simulink model "A1"  (R2023b)
settings: Solver=FixedStepAuto  StartTime=0.0  StopTime=10  FixedStep=1e-3  RelTol=1e-3  EnableMultiTasking=on
undefined symbols (not defined in the file or in its folder): D0, D1, D10, D11, D12, D13, D2, D3, D4, D5, D6, D7, D8, D9, PTA0, PTA1, PTA2, PTB23, PTB9, PTC16, PTC17, PTC2, PTC3, PTC4, PTD0, PTD1, PTD2, PTD3
libraries: frdmk64flib x15
settings Model: PacingRate=0.250000  ExtModeTrigDuration=5  Creator=mathewgaluszka  LastModifiedBy=himan
settings OptimizationCC: EnhancedBackFolding=on  PassReuseOutputArgsAs=Individual arguments  ZeroExternalMemoryAtStartup=off  ZeroInternalMemoryAtStartup=off  MaxStackSize=64  OptimizeBlockOrder=speed  DifferentSizesBufferReuse=on  OptimizationCustomize=off  EfficientTunableParamExpr=on
settings DebuggingCC: ParameterTunabilityLossMsg=error
settings HardwareCC: ProdBitPerPointer=32  ProdBitPerSizeT=32  ProdBitPerPtrDiffT=32  ProdLargestAtomicInteger=Long  ProdLargestAtomicFloat=Double  ProdWordSize=32  ProdHWDeviceType=ARM Compatible->ARM Cortex
settings SFSimCC: MATLABDynamicMemAlloc=off
settings RTWCC: Description=Embedded Coder  SystemTargetFile=ert.tlc  HardwareBoard=NXP FRDM-K64F  TLCOptions="-aInlineSetEventsForThisBaseRateFcn=TLC_FALSE -aSuppressMultiTaskScheduler=TLC_FALSE  -aRateBasedStepFcn=0"  TemplateMakefile=ert_default_tmf  Toolchain=GNU Tools for ARM Embedded Processors
settings CodeAppCC: ForceParamTrailComments=on  IgnoreCustomStorageClasses=off  OperatorAnnotations=on  SimulinkDataObjDesc=on  SFDataObjDesc=on  InsertBlockDesc=on
settings ERTTargetCC: SupportContinuousTime=on  ExtModeTransport=4  ExtModeMexFile=sendToCommService

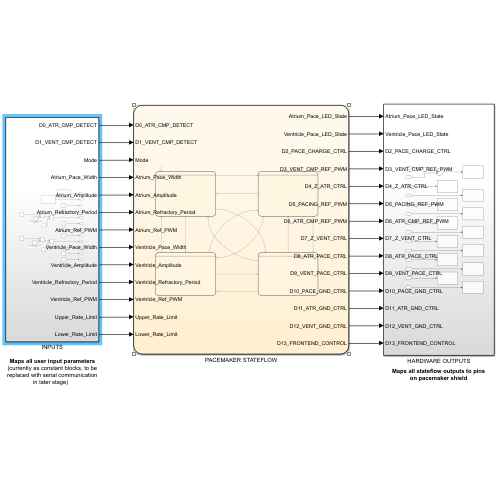
[thumbnail: Simulink's stored preview of the top-level diagram]
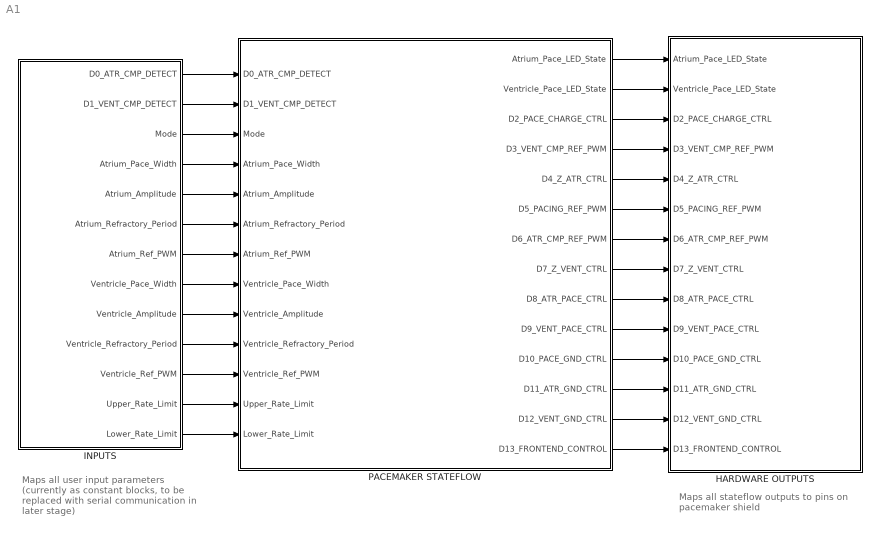
== system A1 ==
  note: Maps all user input parameters (currently as constant blocks, to be replaced with serial communication in later stage)
  note: Maps all stateflow outputs to pins on pacemaker shield
  HARDWARE OUTPUTS : Subsystem
  INPUTS : Subsystem
  PACEMAKER STATEFLOW : Stateflow chart  TreatAsAtomicUnit=on
  wires:
  PACEMAKER STATEFLOW/1(Atrium_Pace_LED_State) -> HARDWARE OUTPUTS/1(Atrium_Pace_LED_State)
  PACEMAKER STATEFLOW/2(Ventricle_Pace_LED_State) -> HARDWARE OUTPUTS/2(Ventricle_Pace_LED_State)
  PACEMAKER STATEFLOW/3(D2_PACE_CHARGE_CTRL) -> HARDWARE OUTPUTS/3(D2_PACE_CHARGE_CTRL)
  PACEMAKER STATEFLOW/4(D3_VENT_CMP_REF_PWM) -> HARDWARE OUTPUTS/4(D3_VENT_CMP_REF_PWM)
  PACEMAKER STATEFLOW/5(D4_Z_ATR_CTRL) -> HARDWARE OUTPUTS/5(D4_Z_ATR_CTRL)
  PACEMAKER STATEFLOW/6(D5_PACING_REF_PWM) -> HARDWARE OUTPUTS/6(D5_PACING_REF_PWM)
  PACEMAKER STATEFLOW/7(D6_ATR_CMP_REF_PWM) -> HARDWARE OUTPUTS/7(D6_ATR_CMP_REF_PWM)
  PACEMAKER STATEFLOW/8(D7_Z_VENT_CTRL) -> HARDWARE OUTPUTS/8(D7_Z_VENT_CTRL)
  PACEMAKER STATEFLOW/9(D8_ATR_PACE_CTRL) -> HARDWARE OUTPUTS/9(D8_ATR_PACE_CTRL)
  PACEMAKER STATEFLOW/10(D9_VENT_PACE_CTRL) -> HARDWARE OUTPUTS/10(D9_VENT_PACE_CTRL)
  PACEMAKER STATEFLOW/11(D10_PACE_GND_CTRL) -> HARDWARE OUTPUTS/11(D10_PACE_GND_CTRL)
  PACEMAKER STATEFLOW/12(D11_ATR_GND_CTRL) -> HARDWARE OUTPUTS/12(D11_ATR_GND_CTRL)
  PACEMAKER STATEFLOW/13(D12_VENT_GND_CTRL) -> HARDWARE OUTPUTS/13(D12_VENT_GND_CTRL)
  PACEMAKER STATEFLOW/14(D13_FRONTEND_CONTROL) -> HARDWARE OUTPUTS/14(D13_FRONTEND_CONTROL)
  INPUTS/1(D0_ATR_CMP_DETECT) -> PACEMAKER STATEFLOW/1(D0_ATR_CMP_DETECT)
  INPUTS/2(D1_VENT_CMP_DETECT) -> PACEMAKER STATEFLOW/2(D1_VENT_CMP_DETECT)
  INPUTS/3(Mode) -> PACEMAKER STATEFLOW/3(Mode)
  INPUTS/4(Atrium_Pace_Width) -> PACEMAKER STATEFLOW/4(Atrium_Pace_Width)
  INPUTS/5(Atrium_Amplitude) -> PACEMAKER STATEFLOW/5(Atrium_Amplitude)
  INPUTS/6(Atrium_Refractory_Period) -> PACEMAKER STATEFLOW/6(Atrium_Refractory_Period)
  INPUTS/7(Atrium_Ref_PWM) -> PACEMAKER STATEFLOW/7(Atrium_Ref_PWM)
  INPUTS/8(Ventricle_Pace_Width) -> PACEMAKER STATEFLOW/8(Ventricle_Pace_Width)
  INPUTS/9(Ventricle_Amplitude) -> PACEMAKER STATEFLOW/9(Ventricle_Amplitude)
  INPUTS/10(Ventricle_Refractory_Period) -> PACEMAKER STATEFLOW/10(Ventricle_Refractory_Period)
  INPUTS/11(Ventricle_Ref_PWM) -> PACEMAKER STATEFLOW/11(Ventricle_Ref_PWM)
  INPUTS/12(Upper_Rate_Limit) -> PACEMAKER STATEFLOW/12(Upper_Rate_Limit)
  INPUTS/13(Lower_Rate_Limit) -> PACEMAKER STATEFLOW/13(Lower_Rate_Limit)

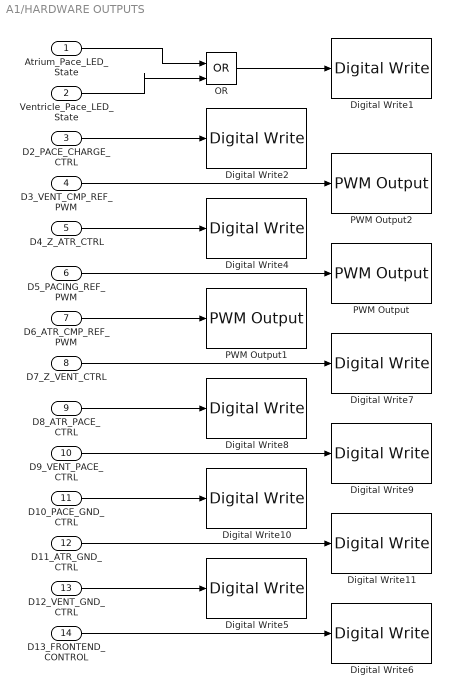
== system A1/HARDWARE OUTPUTS ==
  Atrium_Pace_LED_State : Inport
  Ventricle_Pace_LED_State : Inport  Port=2
  D2_PACE_CHARGE_CTRL : Inport  Port=3
  D3_VENT_CMP_REF_PWM : Inport  Port=4
  D4_Z_ATR_CTRL : Inport  Port=5
  D5_PACING_REF_PWM : Inport  Port=6
  D6_ATR_CMP_REF_PWM : Inport  Port=7
  D7_Z_VENT_CTRL : Inport  Port=8
  D8_ATR_PACE_CTRL : Inport  Port=9
  D9_VENT_PACE_CTRL : Inport  Port=10
  D10_PACE_GND_CTRL : Inport  Port=11
  D11_ATR_GND_CTRL : Inport  Port=12
  D12_VENT_GND_CTRL : Inport  Port=13
  D13_FRONTEND_CONTROL : Inport  Port=14
  Digital Write1 : frdmk64flib/Digital Write  Whichpin=RED_LED
  Digital Write10 : frdmk64flib/Digital Write  Whichpin=PTD0 (D10)
  Digital Write11 : frdmk64flib/Digital Write  Whichpin=PTD2 (D11)
  Digital Write2 : frdmk64flib/Digital Write  Whichpin=PTB9 (D2)
  Digital Write4 : frdmk64flib/Digital Write  Whichpin=PTB23 (D4)
  Digital Write5 : frdmk64flib/Digital Write  Whichpin=PTD3 (D12)
  Digital Write6 : frdmk64flib/Digital Write  Whichpin=PTD1 (D13)
  Digital Write7 : frdmk64flib/Digital Write  Whichpin=PTC3 (D7)
  Digital Write8 : frdmk64flib/Digital Write  Whichpin=PTA0 (D8)
  Digital Write9 : frdmk64flib/Digital Write  Whichpin=PTC4 (D9)
  OR : Logic  Operator=OR  IconShape=distinctive  AllPortsSameDT=off  OutDataTypeStr=boolean
  PWM Output : frdmk64flib/PWM Output  Whichpin=PTA2 (D5)  InitialFrequency=2000  InitialDutyCycle=0
  PWM Output1 : frdmk64flib/PWM Output  Whichpin=PTC2 (D6)  InitialFrequency=2000  InitialDutyCycle=0
  PWM Output2 : frdmk64flib/PWM Output  Whichpin=PTA1 (D3)  InitialFrequency=2000  InitialDutyCycle=0
  wires:
  D2_PACE_CHARGE_CTRL/1 -> Digital Write2/1
  D3_VENT_CMP_REF_PWM/1 -> PWM Output2/1
  D4_Z_ATR_CTRL/1 -> Digital Write4/1
  D5_PACING_REF_PWM/1 -> PWM Output/1
  D6_ATR_CMP_REF_PWM/1 -> PWM Output1/1
  D7_Z_VENT_CTRL/1 -> Digital Write7/1
  D8_ATR_PACE_CTRL/1 -> Digital Write8/1
  D9_VENT_PACE_CTRL/1 -> Digital Write9/1
  D10_PACE_GND_CTRL/1 -> Digital Write10/1
  D11_ATR_GND_CTRL/1 -> Digital Write11/1
  D12_VENT_GND_CTRL/1 -> Digital Write5/1
  D13_FRONTEND_CONTROL/1 -> Digital Write6/1
  Atrium_Pace_LED_State/1 -> OR/1
  Ventricle_Pace_LED_State/1 -> OR/2
  OR/1 -> Digital Write1/1

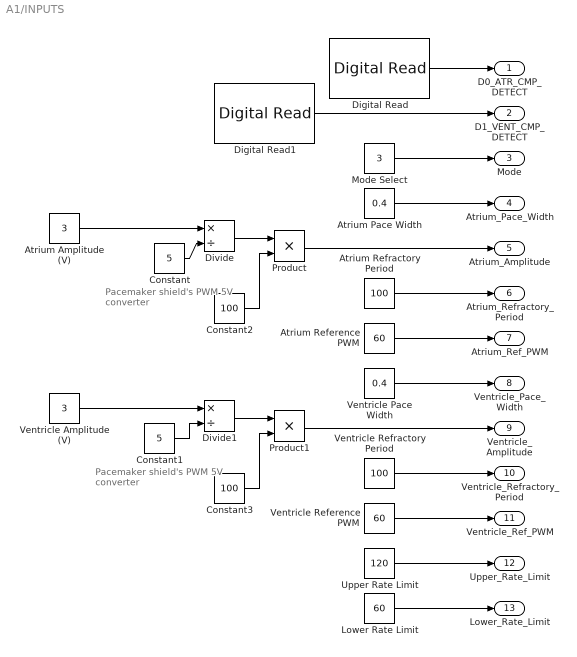
== system A1/INPUTS ==
  note: Pacemaker shield's PWM 5V converter
  note: Pacemaker shield's PWM 5V converter
  Atrium Amplitude (V) : Constant  Value=3
  Atrium Pace Width : Constant  Value=0.4
  Atrium Reference PWM : Constant  Value=60
  Atrium Refractory Period : Constant  Value=100
  Constant : Constant  Value=5
  Constant1 : Constant  Value=5
  Constant2 : Constant  Value=100
  Constant3 : Constant  Value=100
  Digital Read : frdmk64flib/Digital Read  Whichpin=PTC16 (D0)  SampleTime=-1
  Digital Read1 : frdmk64flib/Digital Read  Whichpin=PTC17 (D1)  SampleTime=-1
  Divide : Product  Inputs=*/
  Divide1 : Product  Inputs=*/
  Lower Rate Limit : Constant  Value=60
  Mode Select : Constant  Value=3
  Product : Product
  Product1 : Product
  Upper Rate Limit : Constant  Value=120
  Ventricle Amplitude (V) : Constant  Value=3
  Ventricle Pace Width : Constant  Value=0.4
  Ventricle Reference PWM : Constant  Value=60
  Ventricle Refractory Period : Constant  Value=100
  D0_ATR_CMP_DETECT : Outport
  D1_VENT_CMP_DETECT : Outport  Port=2
  Mode : Outport  Port=3
  Atrium_Pace_Width : Outport  Port=4
  Atrium_Amplitude : Outport  Port=5
  Atrium_Refractory_Period : Outport  Port=6
  Atrium_Ref_PWM : Outport  Port=7
  Ventricle_Pace_Width : Outport  Port=8
  Ventricle_Amplitude : Outport  Port=9
  Ventricle_Refractory_Period : Outport  Port=10
  Ventricle_Ref_PWM : Outport  Port=11
  Upper_Rate_Limit : Outport  Port=12
  Lower_Rate_Limit : Outport  Port=13
  wires:
  Digital Read/1 -> D0_ATR_CMP_DETECT/1
  Digital Read1/1 -> D1_VENT_CMP_DETECT/1
  Mode Select/1 -> Mode/1
  Atrium Pace Width/1 -> Atrium_Pace_Width/1
  Atrium Refractory Period/1 -> Atrium_Refractory_Period/1
  Atrium Reference PWM/1 -> Atrium_Ref_PWM/1
  Ventricle Pace Width/1 -> Ventricle_Pace_Width/1
  Ventricle Refractory Period/1 -> Ventricle_Refractory_Period/1
  Ventricle Reference PWM/1 -> Ventricle_Ref_PWM/1
  Upper Rate Limit/1 -> Upper_Rate_Limit/1
  Lower Rate Limit/1 -> Lower_Rate_Limit/1
  Atrium Amplitude (V)/1 -> Divide/1
  Constant/1 -> Divide/2
  Ventricle Amplitude (V)/1 -> Divide1/1
  Constant1/1 -> Divide1/2
  Divide/1 -> Product/1
  Product/1 -> Atrium_Amplitude/1
  Constant2/1 -> Product/2
  Divide1/1 -> Product1/1
  Product1/1 -> Ventricle_Amplitude/1
  Constant3/1 -> Product1/2

== stateflow chart A1/PACEMAKER STATEFLOW ==
  state AOO
    state Pace
      entry:
      D5_PACING_REF_PWM = 0
      D2_PACE_CHARGE_CTRL=0;
      D10_PACE_GND_CTRL=1;
      D8_ATR_PACE_CTRL=1;
      D11_ATR_GND_CTRL=0;
      D4_Z_ATR_CTRL=0;
      D7_Z_VENT_CTRL=0;
      D12_VENT_GND_CTRL=0;
      D9_VENT_PACE_CTRL=0;
      Atrium_Pace_LED_State=1;
    state Refractory
      entry:
      D10_PACE_GND_CTRL=1;
      D9_VENT_PACE_CTRL=0;
      D4_Z_ATR_CTRL=0;
      D7_Z_VENT_CTRL=0;
      D8_ATR_PACE_CTRL=0;
      D11_ATR_GND_CTRL=1;
      D12_VENT_GND_CTRL=0;
      D2_PACE_CHARGE_CTRL=1;
      D5_PACING_REF_PWM = Atrium_Amplitude
      Atrium_Pace_LED_State=0;
      Standby_Period=(1/(Lower_Rate_Limit))*60000
    (default) -> AOO.Refractory
    AOO.Pace -> AOO.Refractory : [after(Atrium_Pace_Width,msec)]
    AOO.Refractory -> AOO.Pace : [after(Standby_Period,msec)]
  state AAI
    state Refractory
      entry:
      D5_PACING_REF_PWM = Atrium_Amplitude
      D10_PACE_GND_CTRL=1;
      D9_VENT_PACE_CTRL=0;
      D4_Z_ATR_CTRL=0;
      D7_Z_VENT_CTRL=0;
      D8_ATR_PACE_CTRL=0;
      D11_ATR_GND_CTRL=1;
      D12_VENT_GND_CTRL=0;
      D2_PACE_CHARGE_CTRL=1;
      D6_ATR_CMP_REF_PWM = Atrium_Ref_PWM;
      Atrium_Pace_LED_State=0;
      Standby_Period=(1/(Lower_Rate_Limit))*60000-Atrium_Refractory_Period
    state Pace
      entry:
      D5_PACING_REF_PWM = 0
      D2_PACE_CHARGE_CTRL=0;
      D10_PACE_GND_CTRL=1;
      D8_ATR_PACE_CTRL=1;
      D11_ATR_GND_CTRL=0;
      D4_Z_ATR_CTRL=0;
      D7_Z_VENT_CTRL=0;
      D12_VENT_GND_CTRL=0;
      D9_VENT_PACE_CTRL=0;
      Atrium_Pace_LED_State=1;
    (default) -> AAI.Refractory
    AAI.Pace -> (junction 213) : [after(Atrium_Pace_Width,msec)]
    (junction 213) -> AAI.Refractory
    AAI.Refractory -> (junction 213) [order 1] : [D0_ATR_CMP_DETECT == 1]
    (junction 200) -> AAI.Pace [order 2] : after(Standby_Period,msec)
    AAI.Refractory -> (junction 200) [order 2] : [after(Atrium_Refractory_Period,msec) && D0_ATR_CMP_DETECT == 0 ]
    (junction 200) -> AAI.Refractory [order 1] : [D0_ATR_CMP_DETECT == 1]
  state VOO
    state Pace
      entry:
      D5_PACING_REF_PWM = 0
      D2_PACE_CHARGE_CTRL=0;
      D10_PACE_GND_CTRL=1;
      D8_ATR_PACE_CTRL=0;
      D11_ATR_GND_CTRL=0;
      D4_Z_ATR_CTRL=0;
      D7_Z_VENT_CTRL=0;
      D12_VENT_GND_CTRL=0;
      D9_VENT_PACE_CTRL=1;
      Ventricle_Pace_LED_State=1;
    state Refractory
      entry:
      D10_PACE_GND_CTRL=1;
      D9_VENT_PACE_CTRL=0;
      D4_Z_ATR_CTRL=0;
      D7_Z_VENT_CTRL=0;
      D8_ATR_PACE_CTRL=0;
      D11_ATR_GND_CTRL=0;
      D12_VENT_GND_CTRL=1;
      D2_PACE_CHARGE_CTRL=1;
      D5_PACING_REF_PWM = Ventricle_Amplitude
      Ventricle_Pace_LED_State=0;
      Standby_Period=(1/(Lower_Rate_Limit))*60000
    (default) -> VOO.Refractory
    VOO.Pace -> VOO.Refractory : [after(Ventricle_Pace_Width,msec)]
    VOO.Refractory -> VOO.Pace : [after(Standby_Period,msec)]
  state VVI
    state Pace
      entry:
      D5_PACING_REF_PWM = 0
      D2_PACE_CHARGE_CTRL=0;
      D10_PACE_GND_CTRL=1;
      D8_ATR_PACE_CTRL=0;
      D11_ATR_GND_CTRL=0;
      D4_Z_ATR_CTRL=0;
      D7_Z_VENT_CTRL=0;
      D12_VENT_GND_CTRL=0;
      D9_VENT_PACE_CTRL=1;
    state Refractory
      entry:
      D5_PACING_REF_PWM = Ventricle_Amplitude
      D10_PACE_GND_CTRL=1;
      D9_VENT_PACE_CTRL=0;
      D4_Z_ATR_CTRL=0;
      D7_Z_VENT_CTRL=0;
      D8_ATR_PACE_CTRL=0;
      D11_ATR_GND_CTRL=0;
      D12_VENT_GND_CTRL=1;
      D2_PACE_CHARGE_CTRL=1;
      D3_VENT_CMP_REF_PWM = Ventricle_Ref_PWM;
      Ventricle_Pace_LED_State=0;
      Standby_Period=(1/(Lower_Rate_Limit))*60000-Ventricle_Refractory_Period
    (junction 218) -> VVI.Refractory
    VVI.Pace -> (junction 218) : [after(Ventricle_Pace_Width,msec)]
    VVI.Refractory -> (junction 218) [order 1] : [D1_VENT_CMP_DETECT == 1]
    (default) -> VVI.Refractory
    VVI.Refractory -> (junction 219) [order 2] : [after(Ventricle_Refractory_Period,msec) && D1_VENT_CMP_DETECT == 0 ]
    (junction 219) -> VVI.Pace [order 2] : after(Standby_Period,msec)
    (junction 219) -> VVI.Refractory [order 1] : [D1_VENT_CMP_DETECT == 1]
  (default) -> AOO
  AOO -> AAI [order 1] : [Mode==2]
  AAI -> AOO [order 2] : [Mode==0]
  AOO -> VVI [order 3] : [Mode==3]
  VOO -> AAI [order 3] : [Mode==2]
  VOO -> AOO [order 1] : [Mode==0]
  AOO -> VOO [order 2] : [Mode==1]
  VVI -> AOO [order 3] : [Mode==0]
  AAI -> VOO [order 3] : [Mode==1]
  VVI -> AAI [order 2] : [Mode==2]
  AAI -> VVI [order 1] : [Mode==3]
  VOO -> VVI [order 2] : [Mode==3]
  VVI -> VOO [order 1] : [Mode==1]
  data: D0_ATR_CMP_DETECT input; D1_VENT_CMP_DETECT input; Mode input; Atrium_Pace_Width input; Atrium_Amplitude input; Atrium_Refractory_Period input; Atrium_Ref_PWM input; Ventricle_Pace_Width input; Ventricle_Amplitude input; Ventricle_Refractory_Period input; Ventricle_Ref_PWM input; Atrium_Pace_LED_State output; Ventricle_Pace_LED_State output; D2_PACE_CHARGE_CTRL output; D3_VENT_CMP_REF_PWM output; D4_Z_ATR_CTRL output; D5_PACING_REF_PWM output; D6_ATR_CMP_REF_PWM output; D7_Z_VENT_CTRL output; D8_ATR_PACE_CTRL output; D9_VENT_PACE_CTRL output; D10_PACE_GND_CTRL output; D11_ATR_GND_CTRL output; D12_VENT_GND_CTRL output; Upper_Rate_Limit input; Lower_Rate_Limit input; Standby_Period local; D13_FRONTEND_CONTROL output boolean =true
